simulink library "dtlib"  (Simulink 4.00)
undefined symbols (not defined in the file or in its folder): mfread
settings Model: LastModifiedBy=VictorSD

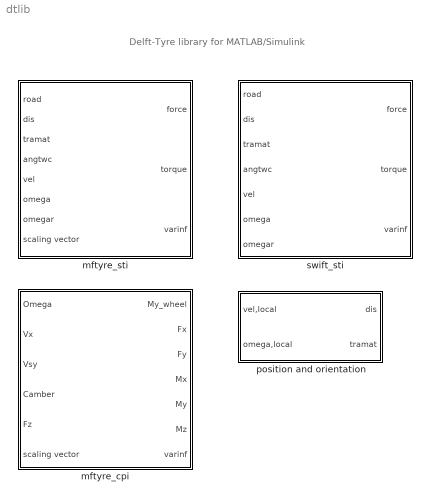
== system dtlib ==
  note: Delft-Tyre library for MATLAB/Simulink
  mftyre_cpi : Subsystem  mask(MFTYRE_CPI){idtyre=1, typarr=mfread('mft_car175_70R13.tir'), use_mode=4}
      mask prompts: idtyre "Tyre ID [integer]"; typarr "TYPARR [double array]"; use_mode "Use mode [integer]"
      mask help:
      | DELFT TYRE Magic Formula for Matlab
      | MF-Tyre 5.2, MF-MCTyre 1.1
      |
      | CONTACT POINT  INTERFACE
      |
      | © 1999-2003 TNO Automotive
      | The Netherlands
      settings: RTWFcnNameOpts=Auto  RTWFileNameOpts=Auto
      mask Help:
      | <!doctype html public "-//w3c//dtd html 4.0 transitional//en">
      | <html>
      | <head>
      |    <meta http-equiv="Content-Type" content="text/html; charset=iso-8859-1">
      |    <meta name="GENERATOR" content="Mozilla/4.72 [en] (X11; I; SunOS 5.7 sun4u) [Netscape]">
      | </head>
      | <body>
      | <font size=+1><b>MFTYRE_CPI: </b>MF-Tyre with Contact Point Interface.</font><p><font size=+1>Calculates tyre forces and moments in the contact point
      | center using the Magic Formula.</font>
      | <br>
      | <hr WIDTH="100%">
      | <br><font size=+1>Inputs:</font>
      | <ul>
      | <li>
      | <b>Omega (1)</b>: wheel angular velocity about wheel spin axis</li>
      | 
      | <li>
      | <b>Vx (1)</b>: forward velocity of wheel center in the wheel plane, parallel
      | to the road surface</li>
      | 
      | <li>
      | <b>Vsy (1)</b>: lateral velocity at road level, parallel to the road surface
      | and perpendicular to the wheel plane</li>
      | 
      | <li>
      | <b>Camber (1)</b>: inclination angle of the wheel with respect to the road</li>
      | 
      | <li>
      | <b>Fz (1)</b>: tyre normal load</li>
      | 
      | <li>
      | <b>scaling vector (7)</b>: contains 7 coefficients to <b>scale</b> the following
      | scaling factors (which are defined in the tyre property file):
      | <br>&nbsp;
      | <br>&nbsp;
      | </li>
      | 
      | <table BORDER WIDTH="60%" NOSAVE >
      | <tr>
      | <td>vector index</td>
      | 
      | <td>scaling factor</td>
      | 
      | <td>scales</td>
      | </tr>
      | 
      | <tr NOSAVE>
      | <td>1</td>
      | 
      | <td>LMUX</td>
      | 
      | <td NOSAVE>peak longitudinal friction coefficient</td>
      | </tr>
      | 
      | <tr>
      | <td>2</td>
      | 
      | <td>LKX</td>
      | 
      | <td>longitudinal slip stiffness</td>
      | </tr>
      | 
      | <tr>
      | <td>3</td>
      | 
      | <td>LMUY</td>
      | 
      | <td>peak lateral friction coefficient</td>
      | </tr>
      | 
      | <tr NOSAVE>
      | <td NOSAVE>4</td>
      | 
      | <td>LKY</td>
      | 
      | <td>cornering stiffness</td>
      | </tr>
      | 
      | <tr>
      | <td>5</td>
      | 
      | <td>LGAY</td>
      | 
      | <td>camber stiffness lateral force</td>
      | </tr>
      | 
      | <tr>
      | <td>6</td>
      | 
      | <td>LTR</td>
      | 
      | <td>pneumatic trail</td>
      | </tr>
      | 
      | <tr>
      | <td>7</td>
      | 
      | <td>LGAZ</td>
      | 
      | <td>camber stiffness aligning moment</td>
      | </tr>
      | </table>
      | 
      | <p><b>NB</b>: The values in the scaling vector <b>do not replace</b> the
      | scaling factors from the tyre property file.
      | <br>The scaling factor that will be used in simulation is the <b>product</b>
      | of the scaling factor in the tyre property
      | <br>file and the corresponding coefficient in the scaling vector.&nbsp;
      | So, if no additional scaling - other than defined
      | <br>in the tyre property file - needs to be applied, a vector of [1 1 1
      | 1 1 1 1] should be used.</ul>
      | 
      | <hr WIDTH="100%">
      | <br><font size=+1>Outputs:</font>
      | <ul>
      | <li>
      | <b>My_wheel (1)</b>: resultant moment about the wheel spin axis</li>
      | 
      | <li>
      | <b>Fx (1)</b>: longitudinal force</li>
      | 
      | <li>
      | <b>Fy (1)</b>: lateral force</li>
      | 
      | <li>
      | <b>Mx (1)</b>: overturning moment</li>
      | 
      | <li>
      | <b>My (1)</b>: rolling resistance moment</li>
      | 
      | <li>
      | <b>Mz (1)</b>: self aligning moment</li>
      | 
      | <li>
      | <b>varinf(40)</b>: extra output variables on tyre behaviour. Most important
      | ones:</li>
      | 
      | <ul>
      | <li>
      | varinf(1): slip angle</li>
      | 
      | <li>
      | varinf(2): longitudinal slip</li>
      | 
      | <li>
      | varinf(3): camber angle</li>
      | 
      | <li>
      | varinf(4..9): Fx, Fy, Fz, Mx, My, Mz</li>
      | 
      | <li>
      | varinf(12): effective rolling radius</li>
      | 
      | <li>
      | varinf(19): longitudinal relaxation length</li>
      | 
      | <li>
      | varinf(20): lateral relaxation length</li>
      | </ul>
      | </ul>
      | 
      | <hr WIDTH="100%">
      | <br><font size=+1>Parameters:</font>
      | 
      | <ul>
      | <li>
      | <b>Tyre ID</b><font size=+1>: </font>integer value which will be printed
      | with messages.</li>
      |     <li><b>TYPARR</b>: variable containing Magic Formula coefficients</li>
      |     <li><b>Use mode</b>: number which defines the operating mode:</li>
      | 
      | &nbsp;<table BORDER WIDTH="60%" NOSAVE >
      | <tr NOSAVE>
      | <td NOSAVE><i>operating mode</i></td>
      | 
      | <td><i>steady-state</i></td>
      | 
      | <td><i>transient</i></td>
      | </tr>
      | 
      | <tr>
      | <td>vertical spring&nbsp;</td>
      | 
      | <td>0</td>
      | 
      | <td>0</td>
      | </tr>
      | 
      | <tr NOSAVE>
      | <td NOSAVE>longitudinal only (Fx, My)</td>
      | 
      | <td>1</td>
      | 
      | <td>11</td>
      | </tr>
      | 
      | <tr>
      | <td>lateral only (Fy, Mx, Mz)</td>
      | 
      | <td>2</td>
      | 
      | <td>12</td>
      | </tr>
      | 
      | <tr>
      | <td>uncombined (Fx, Fy, Mx, My, Mz)</td>
      | 
      | <td>3</td>
      | 
      | <td>13</td>
      | </tr>
      | 
      | <tr>
      | <td>combined (Fx, Fy, Mx, My, Mz)</td>
      | 
      | <td>4</td>
      | 
      | <td>14</td>
      | </tr>
      | </table>
      | 
      | <p><b>NB</b>: for <b>mirrored</b> characteristics, multiply the use mode
      | with '-1'</ul>
      | 
      | <hr WIDTH="100%">
      | <br><font size=+1>General notes:</font>
      | <ul>
      | <li>
      | All calculations are made using SI-units (m, rad, N, kg, s)</li>
      | 
      | <li>
      | The ISO sign convention is adopted for the definitions of slip and tyre
      | force</li>
      | </ul>
      | ©2003 TNO Automotive, Vehicle Dynamics department, The Netherlands
      | </body>
      | </html>
      mask Display:
      | image(imread('dtlogo.jpg','jpg'))
      | 
      | port_label('input',1,'Omega')
      | port_label('input',2,'Vx')
      | port_label('input',3,'Vsy')
      | port_label('input',4,'Camber')
      | port_label('input',5,'Fz')
      | port_label('input',6,'scaling vector')
      | 
      | port_label('output',1,'My_wheel')
      | port_label('output',2,'Fx')
      | port_label('output',3,'Fy')
      | port_label('output',4,'Mx')
      | port_label('output',5,'My')
      | port_label('output',6,'Mz')
      | port_label('output',7,'varinf')
  mftyre_sti : Subsystem  mask(MFTYRE_STI){idtyre=1, typarr=mfread('mft_car175_70R13.tir'), use_mode=4}
      mask prompts: idtyre "Tyre ID [integer]"; typarr "TYPARR [double array]"; use_mode "Use mode [integer]"
      mask help:
      | DELFT TYRE Magic Formula for Matlab
      | MF-Tyre 5.2, MF-MCTyre 1.1
      |
      | STANDARD TYRE INTERFACE (STI 1.4)
      |
      | © 1999-2003 TNO Automotive
      | The Netherlands
      settings: RTWFcnNameOpts=Auto  RTWFileNameOpts=Auto
      mask Help:
      | <!doctype html public "-//w3c//dtd html 4.0 transitional//en">
      | <html>
      | <head>
      |    <meta http-equiv="Content-Type" content="text/html; charset=iso-8859-1">
      |    <meta name="GENERATOR" content="Mozilla/4.72 [en] (X11; I; SunOS 5.7 sun4u) [Netscape]">
      | </head>
      | <body>
      | <font size=+1><b>MFTYRE_STI</b>: MF-Tyre with Standard Tyre Interface</font>
      | <p><font size=+1>Calculates tyre forces and moments in the wheel carrier
      | using the Magic Formula.</font>
      | <p>This block follows the definitions of the Standard Tyre Interface as
      | developed by the TYDEX Workgroup.
      | <br>
      | <hr WIDTH="100%">
      | <br><font size=+1>Inputs:</font>
      | <ul>
      |     <li><b>road (3)</b>: a vector with three components: <br>1- z-value of the
      |     road surface<br>2- dz/dx: slope of the road in x-direction<br>3- dz/dy:
      |     slope of the road in y-direction<br><br>All road data has to be specified
      |     in the global frame. If road undulations are to be included these values
      |     can be made a function of the location of the wheel. The contact algorithm
      |     is not suited for obstacles with a short wavelength and requires that the
      |     z-location of the road be below the wheel center.<br></li>
      |     <li><b>dis (3):</b> a vector with three components: the x, y and z-coordinate
      |     of the wheel carrier in the global axis system.</li>
      |     <li><b>tramat (9):</b> a vector with nine components to specify the transformation
      |     from wheel carrier axis system to the global axis system. Tramat(1..3) is
      |     the representation of the unit x-vector of the carrier axis system in the
      |     global frame. The same applies to tramat(4..6) being the unit y-vector and
      |     tramat(7..9) being the unit z-vector of the carrier axis system expressed
      |     in the global frame.</li>
      |     <li><b>angtwc (1):</b> rotation angle of the wheel with respect to the wheel
      |     carrier about the wheel spin axis (currently not used by MF-Tyre/MF-MCTyre).</li>
      |     <li><b>vel (3):</b> a vector with three components: the global velocity
      |     of the wheel centre expressed in the wheel carrier local frame (x, y and
      |     z component).</li>
      |     <li><b>omega (3):</b> a vector with three components: the global angular
      |     velocity of the wheel centre expressed in the wheel carrier local frame
      |     (x, y and z component).</li>
      |     <li><b>omegar (1):</b> relative angular velocity of the wheel with respect
      |     to the wheel carrier about the wheel spin axis.</li>
      |     <li><b>scaling vector (7)</b>: contains 7 coefficients to scale the following
      |     scaling factors (which are defined in the tyre property file): <br><br></li>
      | </ul>
      | <table border="1" width="430">
      |     <tr>
      |         <td width="47">
      |             <p align="left">vector index&nbsp;</p>
      |         </td>
      |         <td width="95">
      |             <p align="left">&nbsp;scaling factor</p>
      |         </td>
      |         <td width="266">
      |             <p align="left">scales</p>
      |         </td>
      |     </tr>
      |     <tr>
      |         <td width="47">
      |             <p align="left">1</p>
      |         </td>
      |         <td width="95">
      |             <p align="left">LMUX</p>
      |         </td>
      |         <td width="266">
      |             <p align="left">peak longitudinal friction coefficient</p>
      |         </td>
      |     </tr>
      |     <tr>
      |         <td width="47">
      |             <p align="left">2</p>
      |         </td>
      |         <td width="95">
      |             <p align="left">LKX&nbsp;</p>
      |         </td>
      |         <td width="266">
      |             <p align="left">longitudinal slip stiffness</p>
      |         </td>
      |     </tr>
      |     <tr>
      |         <td width="47">
      |             <p align="left">3</p>
      |         </td>
      |         <td width="95">
      |             <p align="left">&nbsp;LMUY</p>
      |         </td>
      |         <td width="266">
      |             <p align="left">peak lateral friction coefficient</p>
      |         </td>
      |     </tr>
      |     <tr>
      |         <td width="47">
      |             <p align="left">4</p>
      |         </td>
      |         <td width="95">
      |             <p align="left">LKY&nbsp;</p>
      |         </td>
      |         <td width="266">
      |             <p align="left">cornering stiffness</p>
      |         </td>
      |     </tr>
      |     <tr>
      |         <td width="47">
      |             <p align="left">5</p>
      |         </td>
      |         <td width="95">
      |             <p align="left">LGAY</p>
      |         </td>
      |         <td width="266">
      |             <p align="left">camber stiffness lateral force</p>
      |         </td>
      |     </tr>
      |     <tr>
      |         <td width="47">
      |             <p align="left">6</p>
      |         </td>
      |         <td width="95">
      |             <p align="left">LTR</p>
      |         </td>
      |         <td width="266">
      |             <p align="left">pneumatic trail</p>
      |         </td>
      |     </tr>
      |     <tr>
      |         <td width="47">
      |             <p align="left">7</p>
      |         </td>
      |         <td width="95">
      |             <p align="left">LGAZ</p>
      |         </td>
      |         <td width="266">
      |             <p align="left">camber stiffness aligning moment</p>
      |         </td>
      |     </tr>
      | </table>
      | <P><b>NB</b>: The values in the scaling vector <b>do not replace</b> the scaling
      | factors from the tyre property file. <BR>The scaling factor that will be used in
      | simulation is the <b>product</b> of the scaling factor in the tyre property
      | <BR>file and the corresponding coefficient in the scaling vector.&nbsp; So, if no
      | additional scaling - other than defined <BR>in the tyre property file - needs to
      | be applied, a vector of [1 1 1 1 1 1 1] should be used.</P><hr WIDTH="100%">
      | <br><font size=+1>Outputs:</font>
      | <ul>
      |     <li><b>force(3):</b> forces applied by the tyre onto the rim at the centre
      |     of the wheel. The force vector has three components in the accompanying
      |     x, y and z direction of the carrier frame.</li>
      |     <li><b>torque(3):</b> moments applied by the tyre onto the rim at the centre
      |     of the wheel, expressed in the carrier axis system. Torque as three components
      |     representing the moments in the x, y and z direction</li>
      |     <li><b>varinf(40)</b>: extra output variables on tyre behaviour. Most important
      | ones:</li>
      | <ul>
      | <li>
      | varinf(1): slip angle</li>
      | 
      | <li>
      | varinf(2): longitudinal slip</li>
      | 
      | <li>
      | varinf(3): camber angle</li>
      | 
      | <li>
      | varinf(4..9): Fx, Fy, Fz, Mx, My, Mz at the tyre contact point</li>
      | 
      | <li>
      | varinf(10): tyre deflection</li>
      | 
      | <li>
      | varinf(11): deflection velocity, normal to the ground</li>
      | 
      | <li>
      | varinf(12): effective rolling radius</li>
      | 
      | <li>
      | varinf(13..15): x, y, z coordinate of the contact point center</li>
      | 
      | <li>
      | varinf(16..18): x, y, z component of the normal to the road</li>
      | 
      | <li>
      | varinf(19): longitudinal relaxation length</li>
      | 
      | <li>
      | varinf(20): lateral relaxation length</li>
      | 
      | <li>
      | varinf(24): longitudinal slip velocity Vsx</li>
      | 
      | <li>
      | varinf(25): lateral slip velocity Vsy</li>
      | 
      | <li>
      | varinf(26): wheel forward velocity Vx</li>
      | </ul>
      | </ul>
      | <hr WIDTH="100%">
      | <br><font size=+1>Parameters:</font>
      | <ul>
      | <li>
      | <b>Tyre ID</b>: integer value which will be printed with messages.</li>
      |     <li><b>TYPARR</b>: variable containing Magic Formula coefficients</li>
      |     <li><b>Use mode</b>: number which defines the operating mode:</li>
      | 
      | &nbsp;<table BORDER WIDTH="60%" NOSAVE >
      | <tr NOSAVE>
      | <td NOSAVE><i>operating mode</i></td>
      | 
      | <td><i>steady-state</i></td>
      | 
      | <td><i>transient</i></td>
      | </tr>
      | 
      | <tr>
      | <td>vertical spring only</td>
      | 
      | <td>0</td>
      | 
      | <td>0</td>
      | </tr>
      | 
      | <tr NOSAVE>
      | <td NOSAVE>longitudinal only (Fx ,My)</td>
      | 
      | <td>1</td>
      | 
      | <td>11</td>
      | </tr>
      | 
      | <tr>
      | <td>lateral only (Fy, Mx, Mz)</td>
      | 
      | <td>2</td>
      | 
      | <td>12</td>
      | </tr>
      | 
      | <tr>
      | <td>uncombined (Fx, Fy, Mx, My, Mz)</td>
      | 
      | <td>3</td>
      | 
      | <td>13</td>
      | </tr>
      | 
      | <tr>
      | <td>combined (Fx, Fy, Mx, My, Mz)</td>
      | 
      | <td>4</td>
      | 
      | <td>14</td>
      | </tr>
      | </table>
      | 
      | <p><b>NB</b>: for <b>mirrored</b> characteristics, multiply the use mode
      | with '-1'
      | <br></ul>
      | 
      | <hr WIDTH="100%">
      | <br><font size=+1>General notes:</font>
      | <ul>
      | <li>
      | All calculations are made using SI-units (m, rad, N, kg, s)</li>
      | 
      | <li>
      | The ISO sign convention is adopted for the definitions of slip and tyre
      | forces</li>
      | </ul>
      | ©2003 TNO Automotive, Vehicle Dynamics department, The Netherlands
      | </body>
      | </html>
      mask Display:
      | image(imread('dtlogo.jpg','jpg'))
      | 
      | port_label('input',1,'road')
      | port_label('input',2,'dis')
      | port_label('input',3,'tramat')
      | port_label('input',4,'angtwc')
      | port_label('input',5,'vel')
      | port_label('input',6,'omega')
      | port_label('input',7,'omegar')
      | port_label('input',8,'scaling vector')
      | 
      | port_label('output',1,'force')
      | port_label('output',2,'torque')
      | port_label('output',3,'varinf')
  position and orientation : Subsystem  mask(Position and Orientation){init_pos=[0 0 0.28], init_angle=[0 0 0]}
      mask prompts: init_pos "Wheel center position (global)"; init_angle "Wheel center orientation (global, Bryant angles, rotation seq. ZXY)"
      mask help:
      | DELFT TYRE Local 2 global transformation for Matlab
      | for use with Standard Tyre Interface (STI).
      |
      | STANDARD TYRE INTERFACE (STI 1.4)
      |
      | © 2002-2003 TNO Automotive
      | The Netherlands
      settings: RTWFcnNameOpts=Auto  RTWFileNameOpts=Auto
      mask Help:
      | <!doctype html public "-//w3c//dtd html 4.0 transitional//en">
      | <html>
      | <head>
      |    <meta http-equiv="Content-Type" content="text/html; charset=iso-8859-1">
      |    <meta name="GENERATOR" content="Mozilla/4.72 [en] (X11; I; SunOS 5.7 sun4u) [Netscape]">
      | </head>
      | <body>
      | <font size=+1><b>Position and orientation</b>: </font><font size="4">Calculation
      | of transformation matrix and global position from local HUB velocities</font>
      | <p><font size="4">Transforms the local translational and angular velocity of
      | the wheel center to the global position and transformation matrix for use with
      | the Standard
      | Tyre Interface (STI)</font></p>
      | <p>This block is supplied as addition for the possible
      | conversion needed to run localized input with MF-Tyre and SWIFT-Tyre implementing
      | the Standard Tyre Interface.<br>
      | <hr WIDTH="100%">
      | <br><font size=+1>Inputs:</font>
      | <ul>
      | <li>
      | <b>vel, &nbsp;local(3)</b>: local velocity of the wheel center expressed in the carrier
      | frame: x, y and z component</li>
      | 
      | <li>
      | <b>omega, local (3)</b>: local  angular velocity of the wheel carrier expressed
      | in the carrier frame: x, y and z component</li>
      | 
      | </ul>
      | 
      | <hr WIDTH="100%">
      | <br><font size=+1>Outputs:</font>
      | <ul>
      | <li>
      | <b>dis(3)</b>: location of the wheel center in the global frame: x, y and z
      | coordinate</li>
      | 
      |     <li><b>tramat(9)</b>: transformation matrix from wheel carrier to the global frame
      | <BR>tramat(1..3): representation of the unit x-vector of the carrier axis in the
      | global frame <BR>tramat(4..6): representation of the unit y-vector of the
      | carrier axis in the global frame <BR>tramat(7..9): representation of the unit
      | z-vector of the carrier axis in the global frame </li>
      | </ul>
      | 
      | <hr WIDTH="100%">
      | <br><font size=+1>Parameters:</font>
      | <ul>
      |     <li>init_pos: Initial wheel center position (global x, y and z
      | coordinate)</li>
      |     <li>init_angle: Initial wheel center orientation (global, Bryant angles, rotation
      |     seq. ZXY)</li>
      | </ul>
      | <hr WIDTH="100%">
      | <br><font size=+1>General notes:</font>
      | <ul>
      | <li>
      | All calculations are made using SI-units (m, rad, N, kg, s)<br>&nbsp;</li>
      | 
      | </ul>
      | ©2003 TNO Automotive, Vehicle Dynamics department, The Netherlands
      | </body>
      | </html>
  swift_sti : Subsystem  mask(SWIFT_STI){idtyre=1, use_mode=24, tpfname='swt_car205_60R15.tir', road_popup=Data file (effective inputs), rdfname='swt_road.rdf'}
      mask prompts: idtyre "Tyre ID [integer]"; use_mode "Use mode [integer]"; tpfname "Tyre property file [string]"; road_popup "Road"; rdfname "Road data file [string]"
      mask help:
      | DELFT TYRE Magic Formula for Matlab
      | SWIFT-Tyre 1.1
      |
      | STANDARD TYRE INTERFACE (STI 1.4)
      |
      | © 2002-2003 TNO Automotive
      | The Netherlands
      mask init:
      | idroad=1;
      | if (road_popup==2)
      |   idroad=100;
      | end
      settings: RTWFcnNameOpts=Auto  RTWFileNameOpts=Auto
      mask Help:
      | <!doctype html public "-//w3c//dtd html 4.0 transitional//en">
      | <html>
      | <head>
      |    <meta http-equiv="Content-Type" content="text/html; charset=iso-8859-1">
      |    <meta name="GENERATOR" content="Mozilla/4.72 [en] (X11; I; SunOS 5.7 sun4u) [Netscape]">
      | </head>
      | <body>
      | <font size=+1><b>SWIFT_STI</b>: SWIFT-Tyre with Standard Tyre Interface</font>
      | <p><font size=+1>Calculates tyre forces and moments in the wheel carrier
      | using SWIFT.</font>
      | <hr WIDTH="100%">
      | <br><font size=+1>Inputs:</font>
      | <ul>
      |     <li><b>road (3)</b>:present for compatibility with MF-Tyre. In SWIFT-Tyre,
      |     the road profile must be defined in an ASCII file format when the check
      |     box 'Effective inputs' is selected. In the road property file the road height
      |     is specified as a function of travelled distance. In a road data file the
      |     left and right track data may be specified; the appropriate track data is
      |     selected depending on the role of the tire in the model. SWIFT uses a zero-order
      |     sample and hold when evaluating the road profile. Changes in the height
      |     of the road profile are interpreted as steps. For maximum accuracy it is
      |     important that the sample points coincide with the data provided by the
      |     user, otherwise interpolated data will be used. So you should use road data
      |     with a fixed sample interval and specify this value for ROAD_INCREMENT in
      |     the [MODEL] section of the tire property file. Typically, the road sample
      |     interval should be in the range of 0.1-0.2 meters or larger.</li>
      | </ul>
      | <ul>
      |     <li>&nbsp;</li>
      |     <li><b>dis (3):</b> a vector with three components: the x, y and z-coordinate
      |     of the wheel carrier in the global axis system.</li>
      |     <li><b>tramat (9):</b> a vector with nine components to specify the transformation
      |     from wheel carrier axis system to the global axis system. Tramat(1..3) is
      |     the representation of the unit x-vector of the carrier axis system in the
      |     global frame. The same applies to tramat(4..6) being the unit y-vector and
      |     tramat(7..9) being the unit z-vector of the carrier axis system expressed
      |     in the global frame.</li>
      |     <li><b>angtwc (1):</b> rotation angle of the wheel with respect to the wheel
      |     carrier about the wheel spin axis.</li>
      |     <li><b>vel (3):</b> a vector with three components: the global velocity
      |     of the wheel centre expressed in the wheel carrier local frame (x, y and
      |     z component).</li>
      |     <li><b>omega (3):</b> a vector with three components: the global angular
      |     velocity of the wheel centre expressed in the wheel carrier local frame
      |     (x, y and z component).</li>
      |     <li><b>omegar (1):</b> relative angular velocity of the wheel with respect
      |     to the wheel carrier about the wheel spin axis.</li>
      | </ul>
      | <hr WIDTH="100%">
      | <br><font size=+1>Outputs:</font>
      | <ul>
      |     <li><b>force(3):</b> forces applied by the tyre onto the rim at the centre
      |     of the wheel. The force vector has three components in the accompanying
      |     x, y and z direction of the carrier frame.</li>
      |     <li><b>torque(3):</b> moments applied by the tyre onto the rim at the centre
      |     of the wheel, expressed in the carrier axis system. Torque as three components
      |     representing the moments in the x, y and z direction</li>
      |     <li><b>varinf(40)</b>: extra output variables on tyre behaviour. Most important
      | ones:</li>
      | <ul>
      | <li>
      | varinf(1): slip angle</li>
      | 
      | <li>
      | varinf(2): longitudinal slip</li>
      | 
      | <li>
      | varinf(3): camber angle</li>
      | 
      | <li>
      | varinf(4..9): Fx, Fy, Fz, Mx, My, Mz at the tyre contact point</li>
      | 
      | <li>
      | varinf(10): tyre deflection</li>
      | 
      | <li>
      | varinf(11): deflection velocity, normal to the ground</li>
      | 
      | <li>
      | varinf(12): effective rolling radius</li>
      | 
      | <li>
      | varinf(13..15): x, y, z coordinate of the contact point center</li>
      | 
      | <li>
      | varinf(16..18): x, y, z component of the normal to the road</li>
      | 
      | <li>
      | varinf(19): longitudinal relaxation length</li>
      | 
      | <li>
      | varinf(20): lateral relaxation length</li>
      | 
      | <li>
      | varinf(24): longitudinal slip velocity Vsx</li>
      | 
      | <li>
      | varinf(25): lateral slip velocity Vsy</li>
      | 
      | <li>
      | varinf(26): wheel forward velocity Vx</li>
      | </ul>
      | </ul>
      | <hr WIDTH="100%">
      | <br><font size=+1>Parameters:</font>
      | <ul>
      |     <li><b>Tyre ID</b> is an integer value identifying the tyre block. This
      |     number will be printed when messages related to the tyre block are printed.
      |     Please take care that the numbers within 1 model are unique. In case effective
      |     inputs is used the following applies: Odd tyre id’s will use the left track
      |     data in the data file &nbsp;while even tyre id’s will use the right track
      |     data from the given data file.</li>
      |     <li><b>Use mode</b> defines the operating mode of the tyre block. See Table
      |     3 of section 2.5.1.<br><br></li>
      | <table BORDER WIDTH="541" NOSAVE >
      | <tr NOSAVE>
      | <td NOSAVE width="252"><i>operating mode</i></td>
      | 
      | <td width="273"><i>SWIFT</i></td>
      | 
      | </tr>
      | 
      | <tr>
      | <td width="252">vertical spring only</td>
      | 
      | <td width="273">20</td>
      | 
      | </tr>
      | 
      | <tr NOSAVE>
      | <td NOSAVE width="252">longitudinal only (Fx ,My)</td>
      | 
      | <td width="273">21</td>
      | 
      | </tr>
      | 
      | <tr>
      | <td width="252">lateral only (Fy, Mx, Mz)</td>
      | 
      | <td width="273">22</td>
      | 
      | </tr>
      | 
      | <tr>
      | <td width="252">uncombined (Fx, Fy, Mx, My, Mz)</td>
      | 
      | <td width="50%">23</td>
      | 
      | </tr>
      | 
      | <tr>
      | <td width="252">combined (Fx, Fy, Mx, My, Mz)</td>
      | 
      | <td width="273">24 (default)</td>
      | 
      | </tr>
      |         <tr>
      | <td width="252">
      |                 <p>mirroring of lateral characteristics</p>
      | </td>
      | 
      | <td width="273">
      |                 <p>Multiply USE_MODE with -1</p>
      | </td>
      | 
      |         </tr>
      |         <tr>
      | <td width="252">
      |                 <p>swift statics</p>
      | </td>
      | 
      | <td width="273">
      |                 <p style="line-height:100%; margin-top:0; margin-bottom:0;">add 100 to positive
      |                 USE_MODE </p>
      |                 <p style="line-height:100%; margin-top:0; margin-bottom:0;">or negate USE_MODE and
      |                 subtract
      |                 100</p>
      | </td>
      | 
      |         </tr>
      | </table>
      | 
      | <p>&nbsp;<li><b>Tyre property file</b> is the file name of the tyre property file
      |     (absolute or relative to current working directory) </li>
      |     <li><b>Road </b>enables you to choose road input via file (Data file (effective
      |     inputs)) or as flat road (external inputs (smooth road).).</li>
      |     <li><b>Road data file</b> contains the file location (absolute or relative
      |     to current working directory) </li>
      | &nbsp;
      | </ul>
      | <hr WIDTH="100%">
      | <br><font size=+1>General notes:</font>
      | <ul>
      | <li>
      | All calculations are made using SI-units (m, rad, N, kg, s)</li>
      | 
      | <li>
      | The ISO sign convention is adopted for the definitions of slip and tyre
      | forces</li>
      | </ul>
      | ©2003 TNO Automotive, Vehicle Dynamics department, The Netherlands
      | </body>
      | </html>
      mask StyleString: edit,edit,edit,popup(External input (smooth road)|Data file (effective inputs)),edit
      mask Display:
      | image(imread('dtlogo.jpg','jpg'))
      | 
      | port_label('input',1,'road')
      | port_label('input',2,'dis')
      | port_label('input',3,'tramat')
      | port_label('input',4,'angtwc')
      | port_label('input',5,'vel')
      | port_label('input',6,'omega')
      | port_label('input',7,'omegar')
      | 
      | port_label('output',1,'force')
      | port_label('output',2,'torque')
      | port_label('output',3,'varinf')

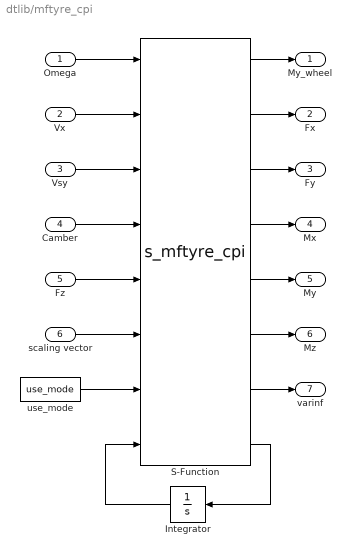
== system dtlib/mftyre_cpi ==
  Omega : Inport  Port=1  LatchInput=off
  Vx : Inport  Port=2  LatchInput=off
  Vsy : Inport  Port=3  LatchInput=off
  Camber : Inport  Port=4  LatchInput=off
  Fz : Inport  Port=5  LatchInput=off
  scaling vector : Inport  Port=6  LatchInput=off
  Integrator : Integrator  Orientation=left  ExternalReset=none  InitialConditionSource=internal  InitialCondition=0  LimitOutput=off  UpperSaturationLimit=inf  LowerSaturationLimit=-inf  ShowSaturationPort=off  ShowStatePort=off  AbsoluteTolerance=auto
  S-Function : S-Function  FunctionName=s_mftyre_cpi  Parameters=idtyre typarr  PortCounts=[]  SFunctionModules=''
  use_mode : Constant  Value=use_mode
  My_wheel : Outport  Port=1
  Fx : Outport  Port=2
  Fy : Outport  Port=3
  Mx : Outport  Port=4
  My : Outport  Port=5
  Mz : Outport  Port=6
  varinf : Outport  Port=7
  wires:
  Integrator/1 -> S-Function/8
  Omega/1 -> S-Function/1
  Vx/1 -> S-Function/2
  Vsy/1 -> S-Function/3
  S-Function/8 -> Integrator/1
  S-Function/7 -> varinf/1
  S-Function/1 -> My_wheel/1
  S-Function/2 -> Fx/1
  S-Function/3 -> Fy/1
  S-Function/4 -> Mx/1
  S-Function/5 -> My/1
  S-Function/6 -> Mz/1
  Camber/1 -> S-Function/4
  Fz/1 -> S-Function/5
  scaling vector/1 -> S-Function/6
  use_mode/1 -> S-Function/7

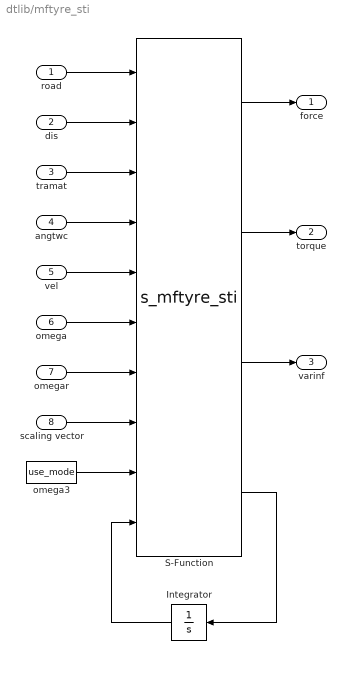
== system dtlib/mftyre_sti ==
  road : Inport  Port=1  LatchInput=off
  dis : Inport  Port=2  LatchInput=off
  tramat : Inport  Port=3  LatchInput=off
  angtwc : Inport  Port=4  LatchInput=off
  vel : Inport  Port=5  LatchInput=off
  omega : Inport  Port=6  LatchInput=off
  omegar : Inport  Port=7  LatchInput=off
  scaling vector : Inport  Port=8  LatchInput=off
  Integrator : Integrator  Orientation=left  ExternalReset=none  InitialConditionSource=internal  InitialCondition=[0 0]  LimitOutput=off  UpperSaturationLimit=inf  LowerSaturationLimit=-inf  ShowSaturationPort=off  ShowStatePort=off  AbsoluteTolerance=auto
  S-Function : S-Function  FunctionName=s_mftyre_sti  Parameters=idtyre typarr  PortCounts=[]  SFunctionModules=''
  omega3 : Constant  Value=use_mode
  force : Outport  Port=1
  torque : Outport  Port=2
  varinf : Outport  Port=3
  wires:
  S-Function/4 -> Integrator/1
  Integrator/1 -> S-Function/10
  S-Function/1 -> force/1
  S-Function/2 -> torque/1
  S-Function/3 -> varinf/1
  omega3/1 -> S-Function/9
  road/1 -> S-Function/1
  omegar/1 -> S-Function/7
  omega/1 -> S-Function/6
  vel/1 -> S-Function/5
  angtwc/1 -> S-Function/4
  tramat/1 -> S-Function/3
  dis/1 -> S-Function/2
  scaling vector/1 -> S-Function/8

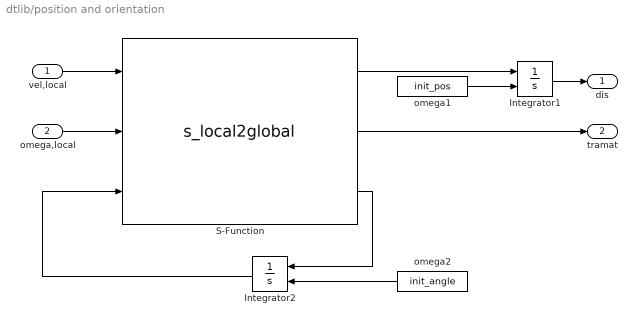
== system dtlib/position and orientation ==
  vel,local : Inport  Port=1  LatchInput=off
  omega,local : Inport  Port=2  LatchInput=off
  Integrator1 : Integrator  ExternalReset=none  InitialConditionSource=external  InitialCondition=0  LimitOutput=off  UpperSaturationLimit=inf  LowerSaturationLimit=-inf  ShowSaturationPort=off  ShowStatePort=off  AbsoluteTolerance=auto
  Integrator2 : Integrator  Orientation=left  ExternalReset=none  InitialConditionSource=external  InitialCondition=0  LimitOutput=off  UpperSaturationLimit=inf  LowerSaturationLimit=-inf  ShowSaturationPort=off  ShowStatePort=off  AbsoluteTolerance=auto
  S-Function : S-Function  FunctionName=s_local2global  PortCounts=[]  SFunctionModules=''
  omega1 : Constant  Value=init_pos
  omega2 : Constant  Orientation=left  Value=init_angle
  dis : Outport  Port=1
  tramat : Outport  Port=2
  wires:
  S-Function/3 -> Integrator2/1
  S-Function/1 -> Integrator1/1
  S-Function/2 -> tramat/1
  Integrator2/1 -> S-Function/3
  omega2/1 -> Integrator2/2
  omega1/1 -> Integrator1/2
  Integrator1/1 -> dis/1
  omega,local/1 -> S-Function/2
  vel,local/1 -> S-Function/1

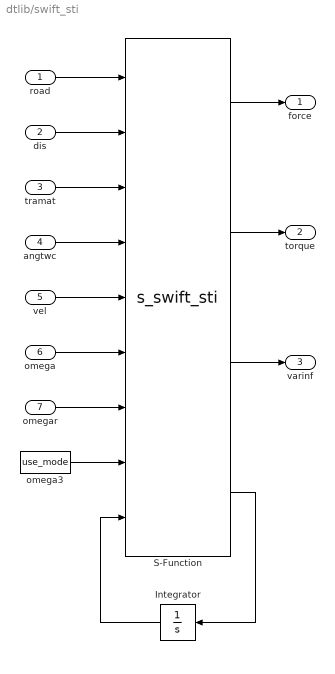
== system dtlib/swift_sti ==
  road : Inport  Port=1  LatchInput=off
  dis : Inport  Port=2  LatchInput=off
  tramat : Inport  Port=3  LatchInput=off
  angtwc : Inport  Port=4  LatchInput=off
  vel : Inport  Port=5  LatchInput=off
  omega : Inport  Port=6  LatchInput=off
  omegar : Inport  Port=7  LatchInput=off
  Integrator : Integrator  Orientation=left  ExternalReset=none  InitialConditionSource=internal  InitialCondition=[0 0 0 0 0 0 0 0 0 0 0 0 0 0 0 0 0 0 0 0 0 0 0 0 0 0 0 0 0 0]  LimitOutput=off  UpperSaturationLimit=inf  LowerSaturationLimit=-inf  ShowSaturationPort=off  ShowStatePort=off  AbsoluteTolerance=auto
  S-Function : S-Function  FunctionName=s_swift_sti  Parameters=idtyre idroad tpfname rdfname  PortCounts=[]  SFunctionModules=''
  omega3 : Constant  Value=use_mode
  force : Outport  Port=1
  torque : Outport  Port=2
  varinf : Outport  Port=3
  wires:
  Integrator/1 -> S-Function/9
  S-Function/4 -> Integrator/1
  omega3/1 -> S-Function/8
  S-Function/1 -> force/1
  S-Function/2 -> torque/1
  S-Function/3 -> varinf/1
  road/1 -> S-Function/1
  omegar/1 -> S-Function/7
  omega/1 -> S-Function/6
  vel/1 -> S-Function/5
  angtwc/1 -> S-Function/4
  tramat/1 -> S-Function/3
  dis/1 -> S-Function/2
